simulink model "sampleModel2005_2"  (R2023a)
settings: Solver=VariableStepAuto  StartTime=0.0  StopTime=10.0  RelTol=1e-3
libraries: hdlsllib x5, simulink x1
settings Model: Creator=user1  LastModifiedBy=user1

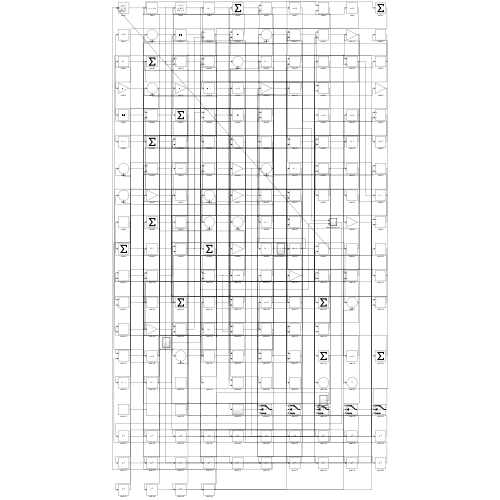
[thumbnail: Simulink's stored preview of the top-level diagram]
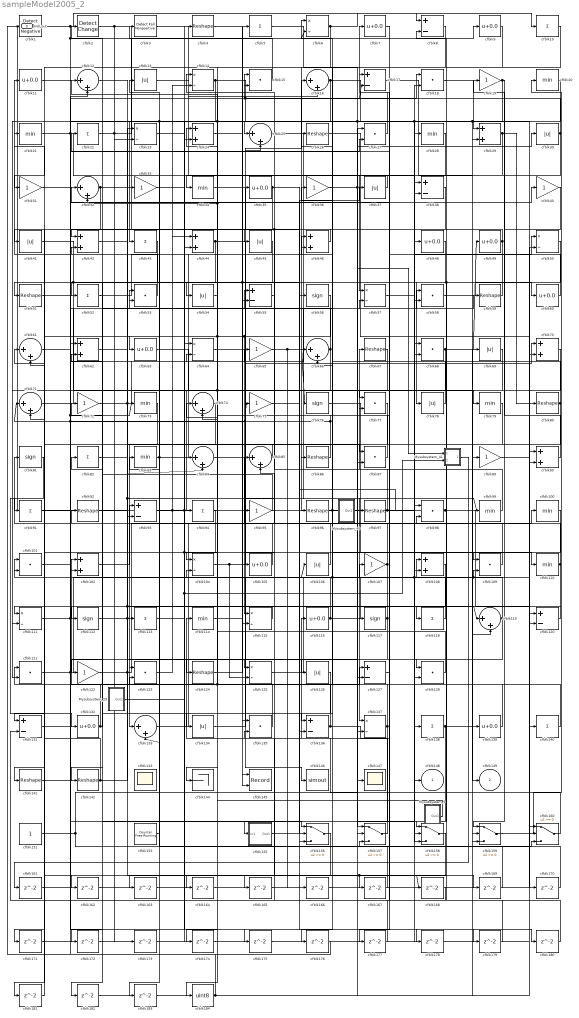
== system sampleModel2005_2 ==
  Mysubsystem_29 : Subsystem  TreatAsAtomicUnit=on  RTWFcnName=Mysubsystem_29
      settings: RTWFcnNameOpts=User specified  RTWFileNameOpts=Use function name
  Mysubsystem_41 : Subsystem  TreatAsAtomicUnit=on  RTWFcnName=Mysubsystem_41
      settings: RTWFcnNameOpts=User specified  RTWFileNameOpts=Use function name
  Mysubsystem_45 : Subsystem  TreatAsAtomicUnit=on  RTWFcnName=Mysubsystem_45
      settings: RTWFcnNameOpts=User specified  RTWFileNameOpts=Use function name
  Mysubsystem_9 : Subsystem  TreatAsAtomicUnit=on  RTWFcnName=Mysubsystem_9
      settings: RTWFcnNameOpts=User specified  RTWFileNameOpts=Use function name
  cfblk1 : hdlsllib/Logic and Bit Operations/Detect Fall Negative  vinit=0  OutDataTypeStr=uint8
  cfblk{5,10,22,43,52,82,91,94,113,118,138,140} (12 alike) : Sum  Inputs=+  OutDataTypeStr=uint8
  cfblk{20..21,28,34,73,79,83,99..100,110,114} (11 alike) : MinMax  OutDataTypeStr=uint8
  cfblk{15,18,27,53,58,68,77,87,98,101,109,121,123,128,135} (15 alike) : DotProduct  OutDataTypeStr=uint8
  cfblk{24,29,42,44,46,62,70,90,102,108} (10 alike) : Sum  OutDataTypeStr=uint8
  cfblk{6,14,23,50,57,64,104,111,115,125,137} (11 alike) : Product  Inputs=*/  OutDataTypeStr=uint8  RndMeth=Zero  SaturateOnIntegerOverflow=on
  cfblk{7,9,11,35,48..49,60,63,105,116,132,139} (12 alike) : Bias  Bias=0.0  SaturateOnIntegerOverflow=off
  cfblk{13,30,37,41,45,54,69,78,106,126,134} (11 alike) : Abs  OutDataTypeStr=uint8  SaturateOnIntegerOverflow=off
  cfblk{19,31,33,36,40,65,72,75,89,95,107,122} (12 alike) : Gain  OutDataTypeStr=uint8
  cfblk{56,76,81,112,117} (5 alike) : Signum
  cfblk{12,16,25,32,61,66,71,74,84..85,119,133} (12 alike) : Sum  Inputs=|++  OutDataTypeStr=uint8
  cfblk{8,17,38,55,93,120,127,131,136} (9 alike) : Sum  Inputs=+-  OutDataTypeStr=uint8
  cfblk{4,26,51,59,67,80,86,92,96..97,124,141..142} (13 alike) : Reshape
  cfblk143 : Scope
      settings: Floating=on
  cfblk144 : Terminator
  cfblk145 : Record  FileSettingsInternal="{\"entries\":[{\"content\":{\"excelSettings\":{\"content\":{},\"type\":\"Streamout.ExcelSettings\"}},\"type\":\"Streamout.FileSettingStorage\",\"uuid\":\"\"}],\"packageUris\":[\"http:\\/\\/schema.mathworks.com\\/mf0\\/streamout_blocks\\/R2020a\"],\"version\":\"1.0\"}"  Layout=[1 1]  SignalsInternal="{\"entries\":[{\"content\":{\"signals\":[{\"content\":{\"blockPath\":[],\"dimensions\":[1],\"domain\":\"\",\"lineColor\":\"#a2142f\",\"plots\":[1],\"port\":1,\"signalID\":57290,\"signalName\":\"cfblk2\"},\"type\":\"RecordBlkView.Signal\",\"uuid\":\"\"},{\"content\":{\"blockPath\":[],\"dimensions\":[1],\"domain\":\"\",\"lineColor\":\"#139fff\",\"plots\":[1],\"port\":2,\"signalID\":57293,\"signalName\":\"cfblk45\"},\"type\":\"RecordBlkView.Signal\",\"uuid\":\"\"}]},\"type\":\"RecordBlkView.InputSignals\",\"uuid\":\"\"}],\"packageUris\":[\"http:\\/\\/schema.mathworks.com\\/mf0\\/streamout_blocks\\/R2020a\"],\"version\":\"1.0\"}"  VisualizationBindings="{\"xyplotplugin\":{\"info\":[{\"series\":[{\"bindingParametersList\":[{\"parameter\":\"X-Axis\",\"signalID\":57290,\"signalName\":\"cfblk2\"},{\"parameter\":\"Y-Axis\",\"signalID\":57293,\"signalName\":\"cfblk45\"}],\"seriesID\":59070}],\"subplotID\":1}]}}"  CompatibilityTag=XY  st=-1
  cfblk146 : ToWorkspace  VariableName=simout  SaveFormat=Timeseries  SampleTime=-1
  cfblk147 : Scope
  cfblk151 : Constant  OutDataTypeStr=uint8  SampleTime=-1
  cfblk153 : hdlsllib/Sources/Counter Free-Running  NumBits=16  tsamp=-1
  cfblk155 : Subsystem
      settings: LibrarySourceBlock=|
      | hdlsllib/Ports &
      | Subsystems/Subsystem
  cfblk{156..160} (5 alike) : Switch  OutDataTypeStr=uint8  SaturateOnIntegerOverflow=off  InputSameDT=off
  cfblk{161..183} (23 alike) : Delay  SampleTime=1
  cfblk184 : DataTypeConversion  OutDataTypeStr=uint8  SaturateOnIntegerOverflow=off  RndMeth=Floor
  cfblk2 : simulink/Logic and Bit Operations/Detect Change  vinit=0  OutDataTypeStr=uint8
      settings: LibrarySourceBlock=|
      | hdlsllib/Logic and Bit
      | Operations/Detect
      | Change
  cfblk3 : hdlsllib/Logic and Bit Operations/Detect Fall Nonpositive  vinit=0  OutDataTypeStr=uint8
  cfblk148 : Outport  OutDataTypeStr=uint8  VectorParamsAs1DForOutWhenUnconnected=off
  cfblk149 : Outport  Port=2  OutDataTypeStr=uint8  VectorParamsAs1DForOutWhenUnconnected=off
  Hdl_out : Outport  Port=3  OutDataTypeStr=uint8
  wires:
  cfblk137/1 -> cfblk102/1, cfblk172/1
  cfblk53/1 -> cfblk11/1
  cfblk123/1 -> cfblk44/1
  cfblk73/1 -> cfblk133/1
  cfblk97/1 -> cfblk67/1, cfblk110/1
  cfblk136/1 -> cfblk32/1, cfblk42/2
  cfblk6/1 -> cfblk31/1, cfblk10/1
  cfblk74/1 -> cfblk142/1
  cfblk8/1 -> cfblk96/1
  cfblk22/1 -> cfblk9/1, cfblk23/2
  cfblk49/1 -> cfblk78/1, cfblk42/1
  cfblk14/1 -> Mysubsystem_41/1(In1), cfblk149/1, cfblk17/2, cfblk43/1
  cfblk25/1 -> cfblk137/1
  cfblk112/1 -> cfblk100/1, cfblk84/2
  cfblk115/1 -> cfblk111/1
  cfblk81/1 -> cfblk132/1
  cfblk29/1 -> cfblk80/1, cfblk66/2
  cfblk87/1 -> cfblk12/1, cfblk32/2
  cfblk11/1 -> cfblk25/1
  cfblk21/1 -> cfblk148/1, cfblk179/1
  cfblk64/1 -> cfblk16/1
  cfblk131/1 -> cfblk58/1
  cfblk125/1 -> cfblk108/1
  cfblk44/1 -> cfblk146/1, cfblk51/1
  cfblk84/1 -> cfblk46/1
  cfblk102/1 -> cfblk93/1
  cfblk66/1 -> cfblk94/1, cfblk2/1
  cfblk37/1 -> cfblk34/1
  cfblk78/1 -> cfblk26/1
  cfblk83/1 -> cfblk25/2, cfblk183/1
  cfblk26/1 -> cfblk140/1
  cfblk134/1 -> cfblk107/1
  cfblk132/1 -> cfblk101/1, cfblk62/2
  cfblk41/1 -> cfblk79/1, cfblk66/1
  cfblk106/1 -> cfblk81/1
  cfblk121/1 -> cfblk27/2, cfblk75/1, cfblk48/1
  cfblk3/1 -> cfblk57/1
  cfblk128/1 -> cfblk74/1
  cfblk33/1 -> cfblk108/2, cfblk117/1
  cfblk85/1 -> cfblk84/1
  cfblk13/1 -> cfblk16/2
  cfblk159/1 -> cfblk20/1
  cfblk104/1 -> cfblk70/1, cfblk125/2
  cfblk52/1 -> cfblk5/1
  cfblk68/1 -> cfblk49/1, cfblk121/2
  cfblk135/1 -> cfblk82/1
  cfblk118/1 -> cfblk21/1
  cfblk160/1 -> cfblk116/1
  cfblk105/1 -> cfblk83/1
  cfblk16/1 -> cfblk144/1, cfblk44/2, cfblk160/2
  cfblk42/1 -> cfblk156/1
  cfblk99/1 -> cfblk14/1
  cfblk65/1 -> cfblk76/1, cfblk166/1
  cfblk67/1 -> cfblk91/1, cfblk134/1
  cfblk138/1 -> cfblk69/1, cfblk165/1
  cfblk56/1 -> cfblk61/2, cfblk174/1, cfblk115/1
  cfblk133/1 -> cfblk85/1
  cfblk43/1 -> cfblk122/1
  cfblk57/1 -> cfblk50/1
  cfblk19/1 -> cfblk111/2, cfblk133/2, cfblk68/2, cfblk109/1
  cfblk109/1 -> cfblk85/2
  cfblk76/1 -> cfblk138/1
  cfblk31/1 -> cfblk45/1
  cfblk24/1 -> cfblk135/1
  cfblk140/1 -> cfblk24/1, cfblk61/1
  cfblk17/1 -> cfblk89/1
  cfblk155/1(Out1) -> cfblk37/1
  cfblk27/1 -> cfblk7/1
  cfblk9/1 -> cfblk54/1
  cfblk111/1 -> cfblk4/1, cfblk18/1, cfblk127/2
  cfblk96/1 -> cfblk139/1, cfblk36/1
  cfblk70/1 -> cfblk93/2
  cfblk80/1 -> cfblk53/2, cfblk171/1
  cfblk69/1 -> cfblk158/1
  cfblk157/1 -> cfblk114/1
  cfblk93/1 -> cfblk167/1, cfblk168/1, cfblk65/1, cfblk14/2
  cfblk98/1 -> cfblk120/2, Hdl_out/1
  cfblk50/1 -> cfblk155/1(In1), cfblk128/1
  cfblk122/1 -> cfblk28/1, cfblk169/1
  cfblk127/1 -> cfblk17/1
  cfblk79/1 -> cfblk95/1
  cfblk117/1 -> cfblk92/1, cfblk156/3
  cfblk114/1 -> cfblk98/2
  cfblk94/1 -> cfblk141/1
  cfblk4/1 -> cfblk38/2
  cfblk116/1 -> cfblk90/2, cfblk18/2, cfblk71/2
  cfblk77/1 -> cfblk136/1
  cfblk71/1 -> cfblk55/1
  cfblk40/1 -> cfblk159/1
  cfblk82/1 -> cfblk87/1
  cfblk54/1 -> cfblk124/1
  cfblk2/1 -> cfblk145/1, cfblk173/1
  cfblk30/1 -> cfblk137/2, cfblk15/2
  cfblk12/1 -> cfblk113/1, cfblk119/1
  cfblk58/1 -> cfblk60/1
  cfblk35/1 -> cfblk63/1, cfblk180/1
  cfblk10/1 -> cfblk86/1
  cfblk59/1 -> cfblk52/1
  cfblk95/1 -> cfblk72/1
  cfblk72/1 -> cfblk57/2, cfblk118/1
  cfblk28/1 -> cfblk158/2
  cfblk51/1 -> cfblk40/1
  cfblk151/1 -> cfblk27/1, cfblk160/3
  cfblk63/1 -> cfblk157/1
  cfblk86/1 -> cfblk15/1, cfblk71/1
  cfblk60/1 -> cfblk22/1
  cfblk100/1 -> cfblk126/1
  cfblk5/1 -> cfblk147/1
  cfblk34/1 -> cfblk56/1
  cfblk124/1 -> cfblk35/1
  cfblk62/1 -> cfblk99/1, cfblk115/2
  cfblk120/1 -> cfblk112/1
  cfblk18/1 -> cfblk29/1
  cfblk107/1 -> cfblk6/1, cfblk104/2
  cfblk90/1 -> cfblk19/1
  cfblk55/1 -> cfblk105/1
  cfblk113/1 -> Mysubsystem_41/2(In2), cfblk59/1
  cfblk91/1 -> cfblk156/2
  cfblk36/1 -> cfblk30/1, cfblk158/3
  cfblk61/1 -> cfblk102/2
  cfblk141/1 -> cfblk127/1
  cfblk119/1 -> cfblk74/2, cfblk109/2, cfblk123/1
  cfblk110/1 -> cfblk53/1, cfblk128/2
  cfblk139/1 -> cfblk106/1, cfblk46/2
  cfblk153/1 -> cfblk13/1
  cfblk46/1 -> cfblk41/1
  cfblk142/1 -> cfblk23/1, cfblk121/1
  cfblk1/1 -> cfblk6/2, cfblk55/2, cfblk8/1
  cfblk15/1 -> cfblk3/1
  cfblk92/1 -> cfblk97/1
  cfblk45/1 -> cfblk145/2, cfblk182/1
  cfblk38/1 -> cfblk125/1, cfblk104/1
  cfblk101/1 -> cfblk64/2, cfblk73/1
  cfblk20/1 -> cfblk77/1, cfblk29/2
  cfblk32/1 -> cfblk131/1, cfblk33/1
  cfblk161/1 -> cfblk12/2
  cfblk126/1 -> cfblk162/1
  cfblk162/1 -> cfblk98/1
  cfblk108/1 -> cfblk163/1
  cfblk163/1 -> cfblk68/1
  cfblk158/1 -> cfblk164/1
  cfblk164/1 -> cfblk120/1
  cfblk165/1 -> cfblk70/2
  cfblk166/1 -> cfblk119/2
  cfblk167/1 -> cfblk123/2
  cfblk168/1 -> cfblk131/2
  cfblk169/1 -> cfblk157/3
  cfblk89/1 -> cfblk170/1
  cfblk170/1 -> cfblk38/1
  cfblk171/1 -> cfblk24/2
  cfblk172/1 -> cfblk58/2
  cfblk173/1 -> cfblk157/2
  cfblk174/1 -> cfblk159/2
  cfblk23/1 -> cfblk175/1
  cfblk175/1 -> cfblk90/1
  cfblk48/1 -> cfblk176/1
  cfblk176/1 -> cfblk1/1
  cfblk7/1 -> cfblk177/1
  cfblk177/1 -> cfblk135/2
  cfblk75/1 -> cfblk178/1
  cfblk178/1 -> cfblk50/2
  cfblk179/1 -> cfblk8/2
  cfblk180/1 -> cfblk77/2
  cfblk156/1 -> cfblk181/1
  cfblk181/1 -> cfblk101/2
  cfblk182/1 -> cfblk160/1
  cfblk183/1 -> cfblk159/3
  cfblk184/1 -> cfblk62/1, cfblk87/2
  Mysubsystem_9/1(Out1) -> cfblk184/1
  Mysubsystem_29/1(Out1) -> cfblk64/1
  Mysubsystem_41/1(Out1) -> cfblk161/1
  Mysubsystem_45/1(Out1) -> cfblk136/2

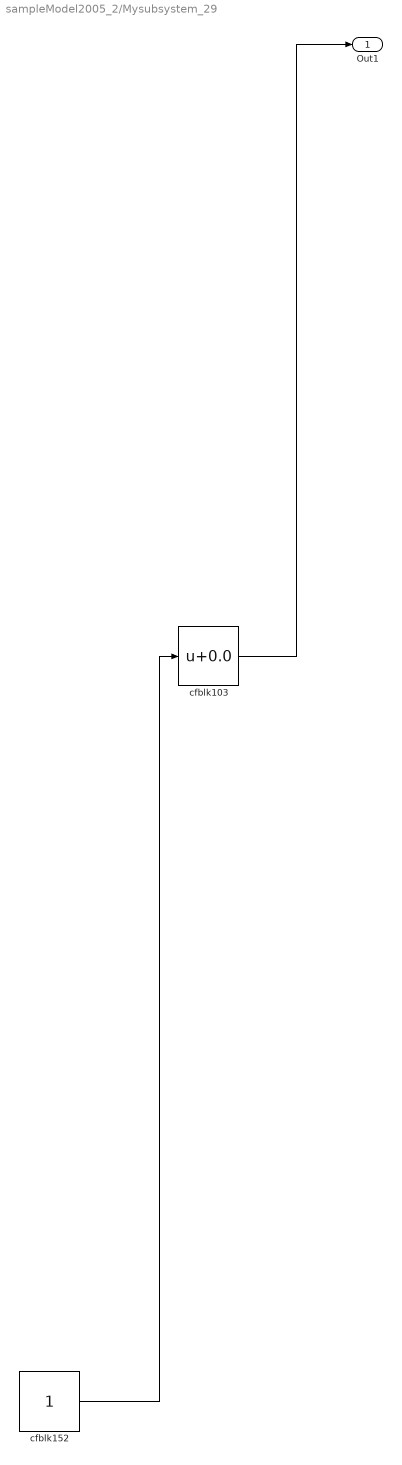
== system sampleModel2005_2/Mysubsystem_29 ==
  cfblk103 : Bias  Bias=0.0  SaturateOnIntegerOverflow=off
  cfblk152 : Constant  SampleTime=-1
  Out1 : Outport
  wires:
  cfblk103/1 -> Out1/1
  cfblk152/1 -> cfblk103/1

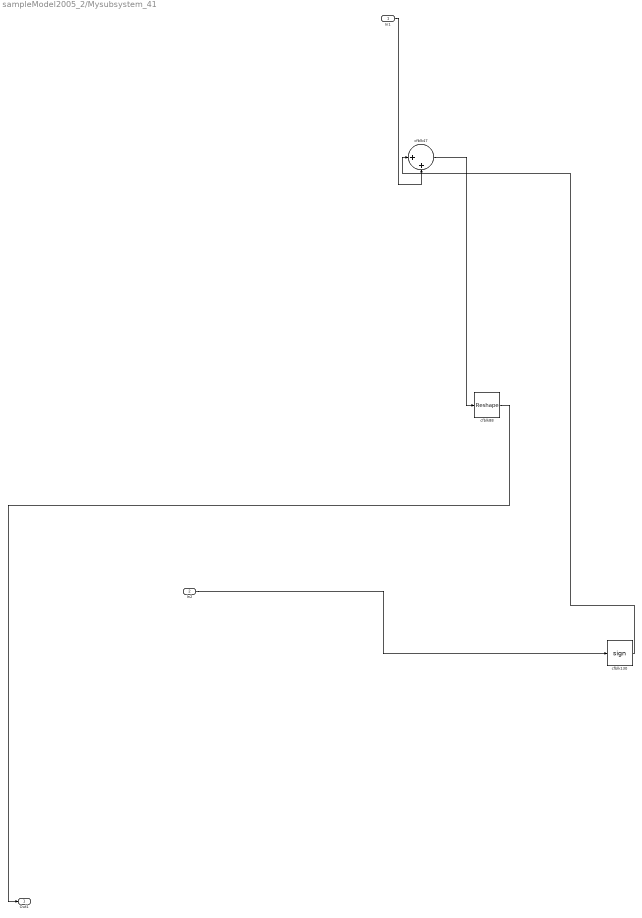
== system sampleModel2005_2/Mysubsystem_41 ==
  In1 : Inport
  In2 : Inport  Port=2
  cfblk130 : Signum
  cfblk47 : Sum  Inputs=|++
  cfblk88 : Reshape
  Out1 : Outport
  wires:
  cfblk130/1 -> cfblk47/1
  cfblk47/1 -> cfblk88/1
  In1/1 -> cfblk47/2
  In2/1 -> cfblk130/1
  cfblk88/1 -> Out1/1

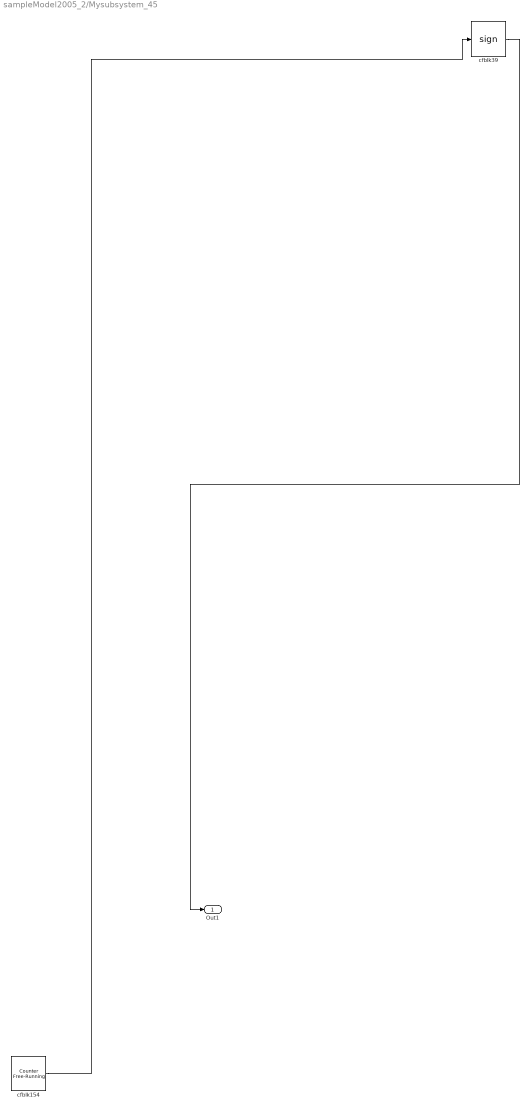
== system sampleModel2005_2/Mysubsystem_45 ==
  cfblk154 : hdlsllib/Sources/Counter Free-Running  NumBits=16  tsamp=-1
  cfblk39 : Signum
  Out1 : Outport
  wires:
  cfblk154/1 -> cfblk39/1
  cfblk39/1 -> Out1/1

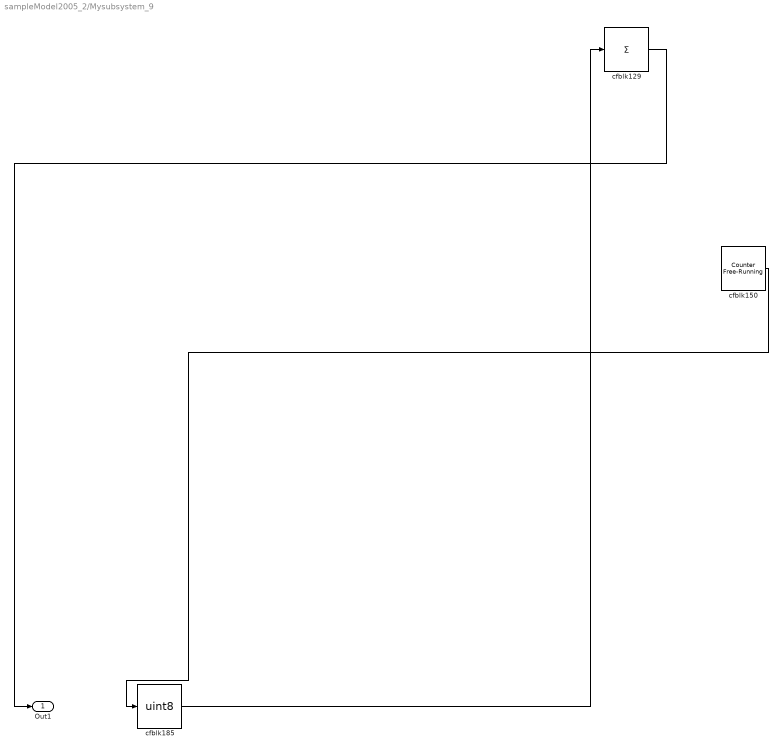
== system sampleModel2005_2/Mysubsystem_9 ==
  cfblk129 : Sum  Inputs=+
  cfblk150 : hdlsllib/Sources/Counter Free-Running  NumBits=16  tsamp=-1
  cfblk185 : DataTypeConversion  OutDataTypeStr=uint8  SaturateOnIntegerOverflow=off  RndMeth=Floor
  Out1 : Outport
  wires:
  cfblk150/1 -> cfblk185/1
  cfblk129/1 -> Out1/1
  cfblk185/1 -> cfblk129/1

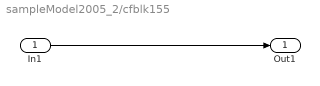
== system sampleModel2005_2/cfblk155 ==
  In1 : Inport
  Out1 : Outport
  wires:
  In1/1 -> Out1/1
